simulink model "HW_PD"  (R2020b)
settings: Solver=FixedStepAuto  StartTime=0.0  StopTime=2  FixedStep=Ts  RelTol=1e-3
undefined symbols (not defined in the file): a_filt, a_sin, b_filt, Kd, Kp, omega_sin, q_0, q_dot_0, q_target
settings Model: Creator=Alberto  LastModifiedBy=Musta

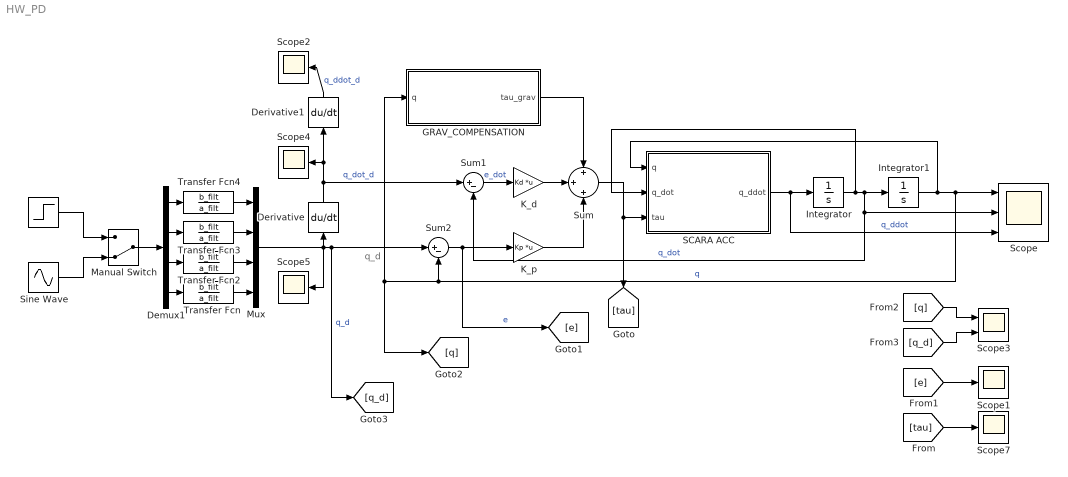
== system HW_PD ==
  note: q_d
  " " : Step  After=q_target  SampleTime=0
  Demux1 : Demux
  Derivative : Derivative
  Derivative1 : Derivative
  GRAV_COMPENSATION : MATLAB Function  TreatAsAtomicUnit=on
  Integrator : Integrator  InitialCondition=q_dot_0
  Integrator1 : Integrator  InitialCondition=q_0
  K_d : Gain  Gain=Kd  Multiplication=Matrix(K*u)
  K_p : Gain  Gain=Kp  Multiplication=Matrix(K*u)
  Manual Switch : ManualSwitch  CurrentSetting=0
  Mux : Mux
  SCARA ACC : MATLAB Function  TreatAsAtomicUnit=on
  Scope : Scope  NumInputPorts=3
  Scope{1..2,4..5,7} (5 alike) : Scope
  Scope3 : Scope  NumInputPorts=2
  Sine Wave : Sin  Amplitude=a_sin  Frequency=omega_sin  SampleTime=0
  Sum : Sum  Inputs=+|+|+
  Sum1 : Sum  Inputs=|+-
  Sum2 : Sum  Inputs=|+-
  Transfer Fcn{,2..4} (4 alike) : TransferFcn  Numerator=b_filt  Denominator=a_filt
  wires:
  SCARA ACC/1(q_ddot) -> Integrator/1, Scope/3  "q_ddot"
  Integrator/1 -> Integrator1/1, Sum1/2, Scope/2, SCARA ACC/2(q_dot)  "q_dot"
  Integrator1/1 -> Scope/1, Sum2/2, [q], GRAV_COMPENSATION/1(q), SCARA ACC/1(q)  "q"
  Demux1/1 -> Transfer Fcn4/1
  Demux1/2 -> Transfer Fcn3/1
  Demux1/3 -> Transfer Fcn2/1
  Demux1/4 -> Transfer Fcn/1
  Transfer Fcn4/1 -> Mux/1
  Transfer Fcn3/1 -> Mux/2
  Transfer Fcn2/1 -> Mux/3
  Transfer Fcn/1 -> Mux/4
  Mux/1 -> Scope5/1, Derivative/1, Sum2/1, [q_d]  "q_d"
  Manual Switch/1 -> Demux1/1
  " "/1 -> Manual Switch/1
  Sine Wave/1 -> Manual Switch/2
  Derivative/1 -> Derivative1/1, Scope4/1, Sum1/1  "q_dot_d"
  Derivative1/1 -> Scope2/1  "q_ddot_d"
  Sum1/1 -> K_d/1  "e_dot"
  Sum/1 -> SCARA ACC/3(tau), [tau]
  K_d/1 -> Sum/2
  Sum2/1 -> [e], K_p/1  "e"
  K_p/1 -> Sum/3
  GRAV_COMPENSATION/1(tau_grav) -> Sum/1
  [q] -> Scope3/1
  [tau] -> Scope7/1
  [e] -> Scope1/1
  [q_d] -> Scope3/2

== matlab function HW_PD/SCARA ACC ==
  data: q input; q_ddot output; q_dot input; tau input
function q_ddot = SCARA_acc(q, q_dot, tau)%#codegen
coder.extrinsic('f_B_mex'); 
coder.extrinsic('f_C_vect_mex'); 
coder.extrinsic('f_g_vect_mex');
B = eye(4);
C_vect = zeros(4,1);
F_g = zeros(4,1);
tau = reshape(tau,4,1);
q_ddot = zeros(4,1);
B = full(f_B_mex('f_B',q));
C_vect = full(f_C_vect_mex('f_C_vect', q, q_dot));
F_g = full(f_g_vect_mex('f_g_vect', q));
q_ddot = (eye(4)/B)*(-C_vect-F_g+tau);

== matlab function HW_PD/GRAV_COMPENSATION ==
  data: q input; tau_grav output
function tau_grav = GRAV_COMPENSATION(q)%#codegen
coder.extrinsic('f_g_vect_mex');
tau_grav = zeros(4,1);
tau_grav = reshape(full(f_g_vect_mex('f_g_vect', q)),4,1);
